simulink library "datacenterCompositeLib"  (R2025b)
settings: Solver=VariableStepAuto  StartTime=0.0  StopTime=10.0  RelTol=1e-3
undefined symbols (not defined in the file): DiscIntNeverNeededParam, ee_sli_rtmsupport, gcbh, Ts, ups
libraries: fl_lib x129, datacenter_lib x32, nesl_utility x16, $bdroot x14, SimscapeFluids_lib x8, simulink x8, eeGeneralControl x6, ee_lib x4, eeTransforms x4, slpidlib x3, eeSinusoidalMeasurementV2 x2, simulink_extras x1
(part 5 of 5)

== system datacenterCompositeLib/Solid State Transformer/PFC Rectifier Controller/Current Controller/Id and Iq Controller/Id Reference Selector ==
  Vmag : Inport
  AND1 : Logic  IconShape=distinctive  AllPortsSameDT=off  OutDataTypeStr=boolean
  Bias : Bias  Bias=0.01  SaturateOnIntegerOverflow=off
  Compare To Constant : simulink/Logic and Bit Operations/Compare To Constant  relop=>  const=0.5  OutDataTypeStr=boolean
  Compare To Constant2 : simulink/Logic and Bit Operations/Compare To Constant  relop=>  const=0.05  OutDataTypeStr=boolean
  Data Type Conversion : DataTypeConversion  SaturateOnIntegerOverflow=off  RndMeth=Floor
  Data Type Conversion1 : DataTypeConversion  OutDataTypeStr=double  SaturateOnIntegerOverflow=off  RndMeth=Floor
  Discrete-Time Integrator : DiscreteIntegrator  IntegratorMethod=Integration: Backward Euler  ExternalReset=falling  SampleTime=ups.sampleTime  LimitOutput=on  UpperSaturationLimit=0.6  LowerSaturationLimit=0  ICPrevOutput=DiscIntNeverNeededParam  ICPrevScaledInput=DiscIntNeverNeededParam
  Mode : Outport
  wires:
  Data Type Conversion/1 -> Mode/1
  Data Type Conversion1/1 -> Discrete-Time Integrator/2, Discrete-Time Integrator/1, AND1/1
  Discrete-Time Integrator/1 -> Compare To Constant2/1
  Compare To Constant2/1 -> AND1/2
  AND1/1 -> Data Type Conversion/1
  Compare To Constant/1 -> Data Type Conversion1/1
  Vmag/1 -> Bias/1
  Bias/1 -> Compare To Constant/1

== system datacenterCompositeLib/Solid State Transformer/PFC Rectifier Controller/DC Voltage Controller and Current Reference/Voltage Controller/Voltage control ==
  e : Inport
  Reset : Inport  Port=2
  Discrete-Time Integrator : DiscreteIntegrator  IntegratorMethod=Integration: Backward Euler  ExternalReset=falling  SampleTime=ups.sampleTime  LimitOutput=on  UpperSaturationLimit=1  LowerSaturationLimit=0  ICPrevOutput=DiscIntNeverNeededParam  ICPrevScaledInput=DiscIntNeverNeededParam
  Ki : Gain  Gain=KiVoltage
  Kp : Gain  Gain=KpVoltage
  Sum7 : Sum  Inputs=|++
  u : Outport  VectorParamsAs1DForOutWhenUnconnected=off
  wires:
  e/1 -> Ki/1, Kp/1
  Ki/1 -> Discrete-Time Integrator/1
  Sum7/1 -> u/1
  Kp/1 -> Sum7/1
  Discrete-Time Integrator/1 -> Sum7/2
  Reset/1 -> Discrete-Time Integrator/2
